simulink model "forwardsim6"  (R2019b)
settings: Solver=FixedStepAuto  StartTime=0.0  StopTime=21.75  FixedStep=1e-2  RelTol=1e-3
undefined symbols (not defined in the file or in its folder): auxdata, DiscIntNeverNeededParam, Earth, forwardsim, struct2bus, WGS84
libraries: aerolibasang x3, aerolibconvert2 x2, sharedutil x2, aerolib6dof2 x1, aerolibatmos2 x1, aerolibgravity2 x1
settings Model: Creator=kieran  LastModifiedBy=kieran

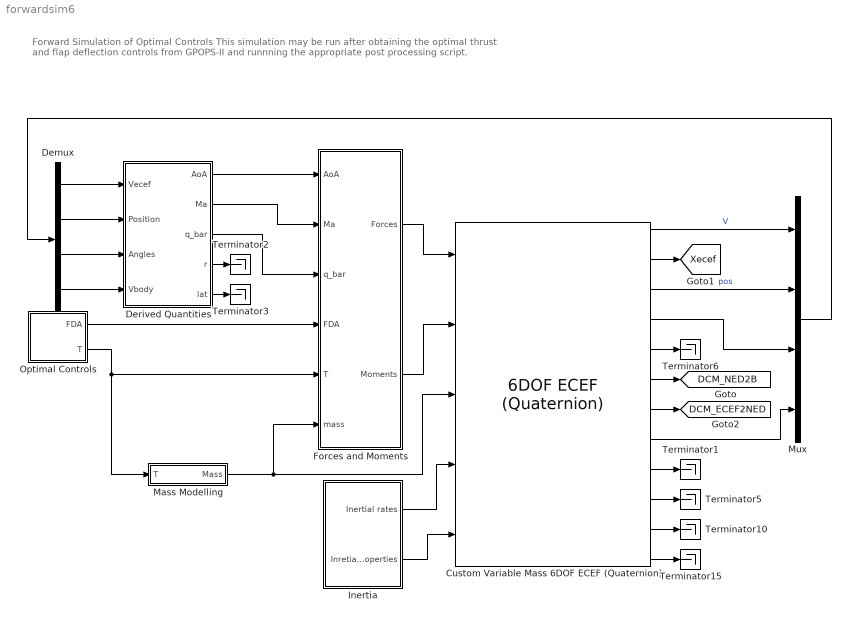
== system forwardsim6 ==
  note: Forward Simulation of Optimal Controls
      | This simulation may be run after obtaining the optimal thrust and flap deflection controls from GPOPS-II and runnning the appropriate post processing script.
  Custom Variable Mass 6DOF ECEF (Quaternion) : aerolib6dof2/6DOF ECEF (Quaternion)  units=Metric (MKS)  mtype=Custom Variable  xg_0=forwardsim.pos0  Vm_0=forwardsim.vel0  eul_0=forwardsim.EO0  pm_0=forwardsim.rot0  mass_0=mass  mass_e=0.5  mass_f=2.0  inertia=inertia  inertia_e=eye(3)  inertia_f=2*eye(3)  vre_flag=off  abi_flag=off  ptype=Earth (WGS84)  R=6378137  F=1/298.257223563  w_E=7292115e-11  angle_in=Internal  LG0=0  quat_statename=''  pm_statename=''  Vm_statename=''  posECEF_statename=''  posECI_statename=''  LG_statename=''  mass_statename=''
      settings: SourceProductName=Aerospace Blockset  SourceProductBaseCode=AE
  Demux : Demux
  Derived Quantities : Subsystem
  Forces and Moments : Subsystem
  Inertia : Subsystem
  Mass Modelling : Subsystem
  Mux : Mux
  Optimal Controls : Subsystem
  Terminator{1..3,5..6,10,15} (7 alike) : Terminator
  tag scope: DCM_ECEF2NED=global, DCM_NED2B=global, Xecef=global
  wires:
  Optimal Controls/2(T) -> Mass Modelling/1(T), Forces and Moments/5(T)
  Mux/1 -> Demux/1
  Inertia/2(Inretial Properties) -> Custom Variable Mass 6DOF ECEF (Quaternion)/5
  Inertia/1(Inertial rates) -> Custom Variable Mass 6DOF ECEF (Quaternion)/4
  Optimal Controls/1(FDA) -> Forces and Moments/4(FDA)
  Mass Modelling/1(Mass) -> Forces and Moments/6(mass), Custom Variable Mass 6DOF ECEF (Quaternion)/3
  Forces and Moments/2(Moments) -> Custom Variable Mass 6DOF ECEF (Quaternion)/2
  Forces and Moments/1(Forces) -> Custom Variable Mass 6DOF ECEF (Quaternion)/1
  Custom Variable Mass 6DOF ECEF (Quaternion)/7 -> [DCM_ECEF2NED]
  Custom Variable Mass 6DOF ECEF (Quaternion)/6 -> [DCM_NED2B]
  Custom Variable Mass 6DOF ECEF (Quaternion)/9 -> Terminator1/1
  Custom Variable Mass 6DOF ECEF (Quaternion)/10 -> Terminator5/1
  Custom Variable Mass 6DOF ECEF (Quaternion)/5 -> Terminator6/1
  Custom Variable Mass 6DOF ECEF (Quaternion)/11 -> Terminator10/1
  Custom Variable Mass 6DOF ECEF (Quaternion)/12 -> Terminator15/1
  Custom Variable Mass 6DOF ECEF (Quaternion)/3 -> Mux/2  "pos"
  Custom Variable Mass 6DOF ECEF (Quaternion)/1 -> Mux/1  "V"
  Custom Variable Mass 6DOF ECEF (Quaternion)/8 -> Mux/4
  Custom Variable Mass 6DOF ECEF (Quaternion)/4 -> Mux/3
  Demux/1 -> Derived Quantities/1(Vecef)
  Demux/2 -> Derived Quantities/2(Position)
  Demux/3 -> Derived Quantities/3(Angles)
  Demux/4 -> Derived Quantities/4(Vbody)
  Derived Quantities/1(AoA) -> Forces and Moments/1(AoA)
  Derived Quantities/2(Ma) -> Forces and Moments/2(Ma)
  Derived Quantities/3(q_bar) -> Forces and Moments/3(q_bar)
  Custom Variable Mass 6DOF ECEF (Quaternion)/2 -> [Xecef]
  Derived Quantities/5(lat) -> Terminator3/1
  Derived Quantities/4(r) -> Terminator2/1

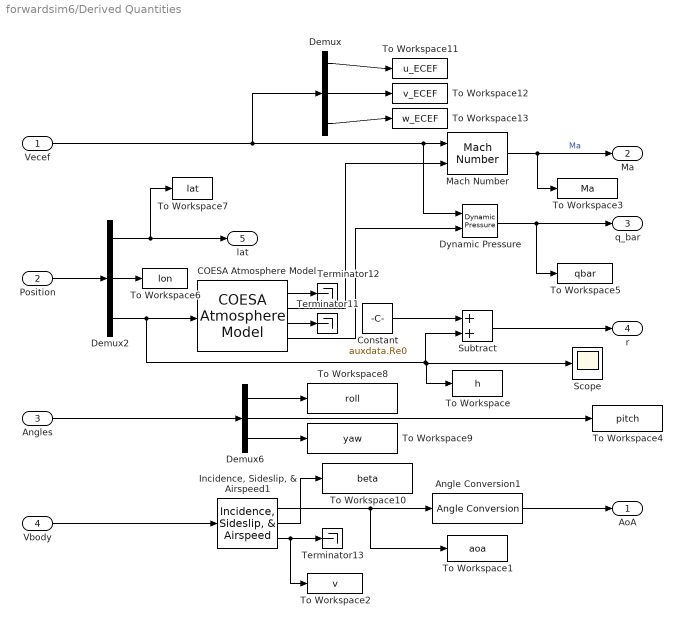
== system forwardsim6/Derived Quantities ==
  Vecef : Inport
  Position : Inport  Port=2
  Angles : Inport  Port=3
  Vbody : Inport  Port=4
  Angle Conversion1 : aerolibconvert2/Angle Conversion  IU=rad  OU=deg
  COESA Atmosphere Model : aerolibatmos2/COESA Atmosphere Model  units=Metric (MKS)  spec=1976 COESA-extended U.S. Standard Atmosphere  model=Profile  profile_var=High temperature  profile_percent=1%  profile_alt=5 km (16404 ft)  envelope_var=High temperature  envelope_percent=1%  action=Warning
  Constant : Constant  Value=auxdata.Re0
  Demux : Demux  Outputs=3
  Demux2 : Demux  Outputs=3
  Demux6 : Demux  Outputs=3
  Dynamic Pressure : aerolibasang/Dynamic Pressure
  "Incidence, Sideslip, & Airspeed1" : aerolibasang/Incidence, Sideslip, & Airspeed
      settings: SourceProductName=Aerospace Blockset
  Mach Number : aerolibasang/Mach Number
      settings: SourceProductName=Aerospace Blockset  SourceProductBaseCode=AE
  Scope : Scope
  Subtract : Sum
  Terminator11 : Terminator
  Terminator12 : Terminator
  Terminator13 : Terminator
  To Workspace : ToWorkspace  VariableName=h  SaveFormat=Timeseries  SampleTime=-1
  To Workspace1 : ToWorkspace  VariableName=aoa  SaveFormat=Timeseries  SampleTime=-1
  To Workspace10 : ToWorkspace  VariableName=beta  SaveFormat=Timeseries  SampleTime=-1
  To Workspace11 : ToWorkspace  VariableName=u_ECEF  SaveFormat=Timeseries  SampleTime=-1
  To Workspace12 : ToWorkspace  VariableName=v_ECEF  SaveFormat=Timeseries  SampleTime=-1
  To Workspace13 : ToWorkspace  VariableName=w_ECEF  SaveFormat=Timeseries  SampleTime=-1
  To Workspace2 : ToWorkspace  VariableName=v  SaveFormat=Timeseries  SampleTime=-1
  To Workspace3 : ToWorkspace  VariableName=Ma  SaveFormat=Timeseries  SampleTime=-1
  To Workspace4 : ToWorkspace  VariableName=pitch  SaveFormat=Timeseries  SampleTime=-1
  To Workspace5 : ToWorkspace  VariableName=qbar  SaveFormat=Timeseries  SampleTime=-1
  To Workspace6 : ToWorkspace  VariableName=lon  SaveFormat=Timeseries  SampleTime=-1
  To Workspace7 : ToWorkspace  VariableName=lat  SaveFormat=Timeseries  SampleTime=-1
  To Workspace8 : ToWorkspace  VariableName=roll  SaveFormat=Timeseries  SampleTime=-1
  To Workspace9 : ToWorkspace  VariableName=yaw  SaveFormat=Timeseries  SampleTime=-1
  AoA : Outport
  Ma : Outport  Port=2
  q_bar : Outport  Port=3
  r : Outport  Port=4
  lat : Outport  Port=5
  wires:
  Demux2/2 -> To Workspace6/1
  COESA Atmosphere Model/3 -> Terminator11/1
  Vecef/1 -> Demux/1, Dynamic Pressure/1, Mach Number/1
  "Incidence, Sideslip, & Airspeed1"/2 -> To Workspace10/1
  COESA Atmosphere Model/1 -> Terminator12/1
  Demux2/3 -> To Workspace/1, Scope/1, Subtract/2, COESA Atmosphere Model/1
  Demux2/1 -> To Workspace7/1, lat/1
  COESA Atmosphere Model/2 -> Mach Number/2
  Demux6/3 -> To Workspace9/1
  Angles/1 -> Demux6/1
  Subtract/1 -> r/1
  COESA Atmosphere Model/4 -> Dynamic Pressure/2
  "Incidence, Sideslip, & Airspeed1"/3 -> Terminator13/1, To Workspace2/1
  "Incidence, Sideslip, & Airspeed1"/1 -> To Workspace1/1, Angle Conversion1/1
  Vbody/1 -> "Incidence, Sideslip, & Airspeed1"/1
  Demux6/1 -> To Workspace8/1
  Position/1 -> Demux2/1
  Angle Conversion1/1 -> AoA/1
  Mach Number/1 -> To Workspace3/1, Ma/1  "Ma"
  Dynamic Pressure/1 -> To Workspace5/1, q_bar/1
  Demux6/2 -> To Workspace4/1
  Constant/1 -> Subtract/1
  Demux/1 -> To Workspace11/1
  Demux/3 -> To Workspace13/1
  Demux/2 -> To Workspace12/1

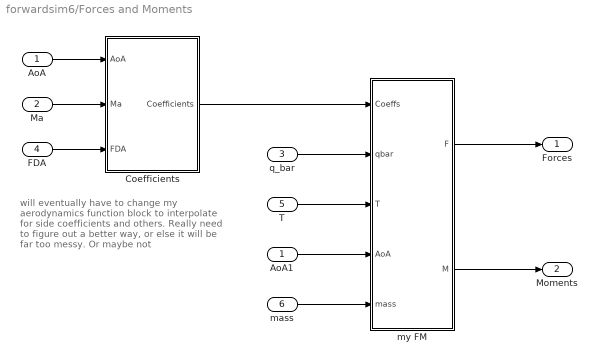
== system forwardsim6/Forces and Moments ==
  note: will eventually have to change my aerodynamics function block to interpolate for side coefficients and others. Really need to figure out a better way, or else it will be far too messy.
      |
      | Or maybe not
  AoA : Inport
  Ma : Inport  Port=2
  q_bar : Inport  Port=3
  FDA : Inport  Port=4
  T : Inport  Port=5
  mass : Inport  Port=6
  AoA1 : InportShadow
  Coefficients : Subsystem
  my FM : Subsystem
  Forces : Outport
  Moments : Outport  Port=2
  wires:
  Ma/1 -> Coefficients/2(Ma)
  FDA/1 -> Coefficients/3(FDA)
  Coefficients/1(Coefficients) -> my FM/1(Coeffs)
  q_bar/1 -> my FM/2(qbar)
  T/1 -> my FM/3(T)
  AoA/1 -> Coefficients/1(AoA)
  my FM/1(F) -> Forces/1
  AoA1/1 -> my FM/4(AoA)
  mass/1 -> my FM/5(mass)
  my FM/2(M) -> Moments/1

== system forwardsim6/Inertia ==
  Constant : Constant  Value=auxdata.MOI
  Constant3 : Constant  Commented=on  Value=auxdata.Iyy
  Inertia : Subsystem  Commented=on
  Inertial Rates : Subsystem
  Inertial rates : Outport
  Inretial Properties : Outport  Port=2
  wires:
  Constant3/1 -> Inertia/1(In1)
  Inertial Rates/1(Out1) -> Inertial rates/1
  Constant/1 -> Inretial Properties/1

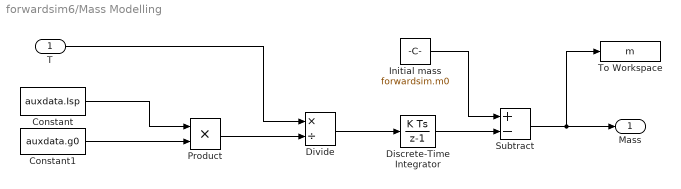
== system forwardsim6/Mass Modelling ==
  T : Inport
  Constant : Constant  Value=auxdata.Isp
  Constant1 : Constant  Value=auxdata.g0
  Discrete-Time Integrator : DiscreteIntegrator  SampleTime=-1  ICPrevOutput=DiscIntNeverNeededParam  ICPrevScaledInput=DiscIntNeverNeededParam
  Divide : Product  Inputs=*/
  Initial mass : Constant  Value=forwardsim.m0
  Product : Product
  Subtract : Sum  Inputs=+-
  To Workspace : ToWorkspace  VariableName=m  SaveFormat=Timeseries  SampleTime=-1
  Mass : Outport
  wires:
  Constant1/1 -> Product/2
  Divide/1 -> Discrete-Time Integrator/1
  Product/1 -> Divide/2
  Constant/1 -> Product/1
  Subtract/1 -> To Workspace/1, Mass/1
  Discrete-Time Integrator/1 -> Subtract/2
  Initial mass/1 -> Subtract/1
  T/1 -> Divide/1

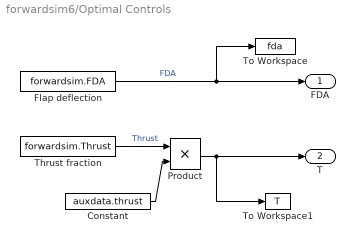
== system forwardsim6/Optimal Controls ==
  Constant : Constant  Value=auxdata.thrust
  Flap deflection : FromWorkspace  VariableName=forwardsim.FDA  SampleTime=0
  Product : Product
  Thrust fraction : FromWorkspace  VariableName=forwardsim.Thrust  SampleTime=0
  To Workspace : ToWorkspace  VariableName=fda  SaveFormat=Timeseries  SampleTime=-1
  To Workspace1 : ToWorkspace  VariableName=T  SaveFormat=Timeseries  SampleTime=-1
  FDA : Outport
  T : Outport  Port=2
  wires:
  Flap deflection/1 -> To Workspace/1, FDA/1  "FDA"
  Constant/1 -> Product/2
  Product/1 -> T/1, To Workspace1/1
  Thrust fraction/1 -> Product/1  "Thrust"

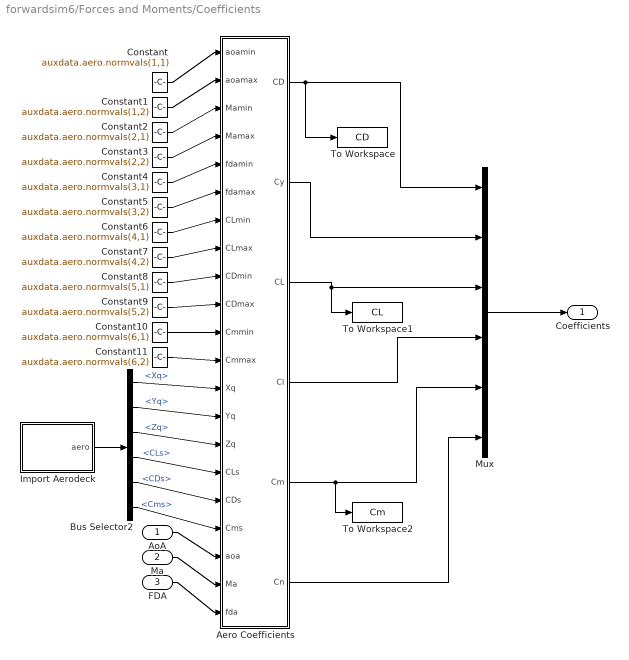
== system forwardsim6/Forces and Moments/Coefficients ==
  AoA : Inport
  Ma : Inport  Port=2
  FDA : Inport  Port=3
  Aero Coefficients : MATLAB Function  TreatAsAtomicUnit=on
  Bus Selector2 : BusSelector  OutputSignals=Xq,Yq,Zq,CLs,CDs,Cms
  Constant : Constant  Value=auxdata.aero.normvals(1,1)
  Constant1 : Constant  Value=auxdata.aero.normvals(1,2)
  Constant10 : Constant  Value=auxdata.aero.normvals(6,1)
  Constant11 : Constant  Value=auxdata.aero.normvals(6,2)
  Constant2 : Constant  Value=auxdata.aero.normvals(2,1)
  Constant3 : Constant  Value=auxdata.aero.normvals(2,2)
  Constant4 : Constant  Value=auxdata.aero.normvals(3,1)
  Constant5 : Constant  Value=auxdata.aero.normvals(3,2)
  Constant6 : Constant  Value=auxdata.aero.normvals(4,1)
  Constant7 : Constant  Value=auxdata.aero.normvals(4,2)
  Constant8 : Constant  Value=auxdata.aero.normvals(5,1)
  Constant9 : Constant  Value=auxdata.aero.normvals(5,2)
  Import Aerodeck : MATLAB Function  InitFcn=struct2bus(auxdata.aero,'aerodeck')  TreatAsAtomicUnit=on
  Mux : Mux  Inputs=6
  To Workspace : ToWorkspace  VariableName=CD  SaveFormat=Timeseries  SampleTime=-1
  To Workspace1 : ToWorkspace  VariableName=CL  SaveFormat=Timeseries  SampleTime=-1
  To Workspace2 : ToWorkspace  VariableName=Cm  SaveFormat=Timeseries  SampleTime=-1
  Coefficients : Outport
  wires:
  Bus Selector2/1 -> Aero Coefficients/13(Xq)  "<Xq>"
  Constant11/1 -> Aero Coefficients/12(Cmmax)
  Bus Selector2/3 -> Aero Coefficients/15(Zq)  "<Zq>"
  Aero Coefficients/5(Cm) -> Mux/5, To Workspace2/1
  Mux/1 -> Coefficients/1
  Aero Coefficients/2(Cy) -> Mux/2
  Constant3/1 -> Aero Coefficients/4(Mamax)
  Constant1/1 -> Aero Coefficients/2(aoamax)
  Constant5/1 -> Aero Coefficients/6(fdamax)
  Constant4/1 -> Aero Coefficients/5(fdamin)
  Constant8/1 -> Aero Coefficients/9(CDmin)
  AoA/1 -> Aero Coefficients/19(aoa)
  Constant7/1 -> Aero Coefficients/8(CLmax)
  FDA/1 -> Aero Coefficients/21(fda)
  Bus Selector2/5 -> Aero Coefficients/17(CDs)  "<CDs>"
  Aero Coefficients/3(CL) -> Mux/3, To Workspace1/1
  Constant2/1 -> Aero Coefficients/3(Mamin)
  Constant10/1 -> Aero Coefficients/11(Cmmin)
  Constant9/1 -> Aero Coefficients/10(CDmax)
  Aero Coefficients/1(CD) -> Mux/1, To Workspace/1
  Constant6/1 -> Aero Coefficients/7(CLmin)
  Import Aerodeck/1(aero) -> Bus Selector2/1
  Bus Selector2/6 -> Aero Coefficients/18(Cms)  "<Cms>"
  Ma/1 -> Aero Coefficients/20(Ma)
  Aero Coefficients/6(Cn) -> Mux/6
  Bus Selector2/4 -> Aero Coefficients/16(CLs)  "<CLs>"
  Constant/1 -> Aero Coefficients/1(aoamin)
  Bus Selector2/2 -> Aero Coefficients/14(Yq)  "<Yq>"
  Aero Coefficients/4(Cl) -> Mux/4

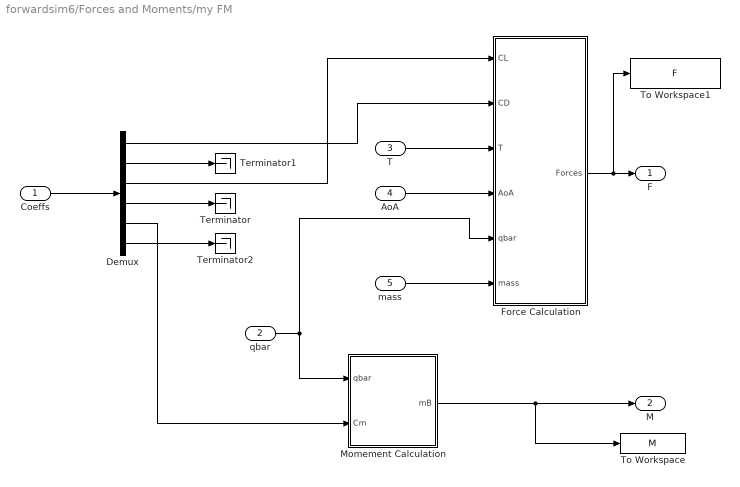
== system forwardsim6/Forces and Moments/my FM ==
  Coeffs : Inport
  qbar : Inport  Port=2
  T : Inport  Port=3
  AoA : Inport  Port=4
  mass : Inport  Port=5
  Demux : Demux  Outputs=6
  Force Calculation : Subsystem
  Momement Calculation : Subsystem
  Terminator : Terminator
  Terminator1 : Terminator
  Terminator2 : Terminator
  To Workspace : ToWorkspace  VariableName=M  SaveFormat=Timeseries  SampleTime=-1
  To Workspace1 : ToWorkspace  VariableName=F  SaveFormat=Timeseries  SampleTime=-1
  F : Outport
  M : Outport  Port=2
  wires:
  Coeffs/1 -> Demux/1
  Demux/5 -> Momement Calculation/2(Cm)
  Demux/4 -> Terminator/1
  Demux/2 -> Terminator1/1
  Demux/6 -> Terminator2/1
  qbar/1 -> Force Calculation/5(qbar), Momement Calculation/1(qbar)
  T/1 -> Force Calculation/3(T)
  AoA/1 -> Force Calculation/4(AoA)
  Force Calculation/1(Forces) -> To Workspace1/1, F/1
  Momement Calculation/1(mB) -> To Workspace/1, M/1
  Demux/1 -> Force Calculation/2(CD)
  Demux/3 -> Force Calculation/1(CL)
  mass/1 -> Force Calculation/6(mass)

== system forwardsim6/Inertia/Inertia ==
  In1 : Inport
  Constant : Constant  Value=0
  Constant1 : Constant  Value=0
  Create 3x3 Matrix : sharedutil/Create 3x3 Matrix  aMode=aMode
  Out1 : Outport
  wires:
  Create 3x3 Matrix/1 -> Out1/1
  Constant/1 -> Create 3x3 Matrix/2, Create 3x3 Matrix/3, Create 3x3 Matrix/4
  Constant1/1 -> Create 3x3 Matrix/8, Create 3x3 Matrix/6, Create 3x3 Matrix/7
  In1/1 -> Create 3x3 Matrix/1, Create 3x3 Matrix/9, Create 3x3 Matrix/5

== system forwardsim6/Inertia/Inertial Rates ==
  Constant1 : Constant  Value=0
  Create 3x3 Matrix : sharedutil/Create 3x3 Matrix  aMode=aMode
  Out1 : Outport
  wires:
  Create 3x3 Matrix/1 -> Out1/1
  Constant1/1 -> Create 3x3 Matrix/1, Create 3x3 Matrix/2, Create 3x3 Matrix/3, Create 3x3 Matrix/4, Create 3x3 Matrix/9, Create 3x3 Matrix/8, Create 3x3 Matrix/7, Create 3x3 Matrix/6, Create 3x3 Matrix/5

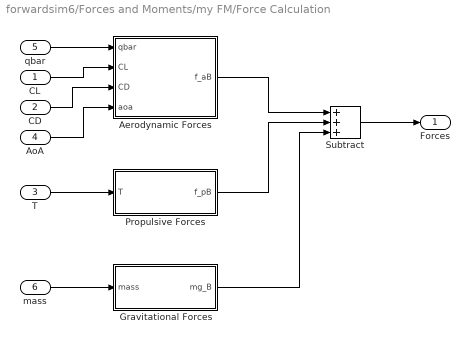
== system forwardsim6/Forces and Moments/my FM/Force Calculation ==
  CL : Inport
  CD : Inport  Port=2
  T : Inport  Port=3
  AoA : Inport  Port=4
  qbar : Inport  Port=5
  mass : Inport  Port=6
  Aerodynamic Forces : Subsystem
  Gravitational Forces : Subsystem
  Propulsive Forces : Subsystem
  Subtract : Sum  Inputs=+++
  Forces : Outport
  wires:
  AoA/1 -> Aerodynamic Forces/4(aoa)
  Aerodynamic Forces/1(f_aB) -> Subtract/1
  Propulsive Forces/1(f_pB) -> Subtract/2
  qbar/1 -> Aerodynamic Forces/1(qbar)
  CL/1 -> Aerodynamic Forces/2(CL)
  CD/1 -> Aerodynamic Forces/3(CD)
  T/1 -> Propulsive Forces/1(T)
  mass/1 -> Gravitational Forces/1(mass)
  Subtract/1 -> Forces/1
  Gravitational Forces/1(mg_B) -> Subtract/3

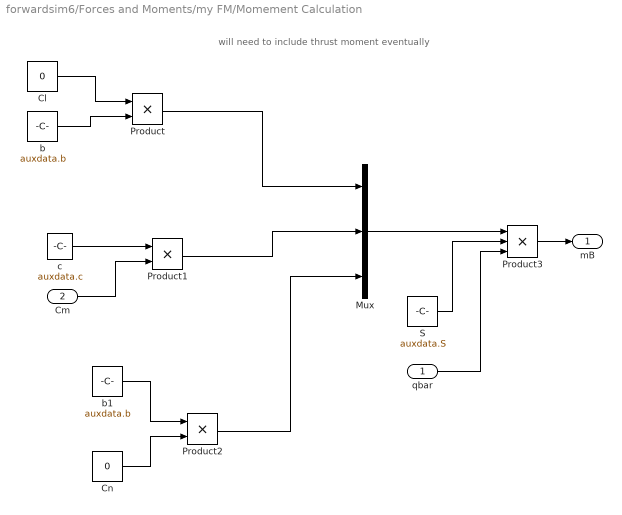
== system forwardsim6/Forces and Moments/my FM/Momement Calculation ==
  note: will need to include thrust moment eventually
  qbar : Inport
  Cm : Inport  Port=2
  Cl : Constant  Value=0
  Cn : Constant  Value=0
  Mux : Mux  Inputs=3
  Product : Product
  Product1 : Product
  Product2 : Product
  Product3 : Product  Inputs=3
  S : Constant  Value=auxdata.S
  b : Constant  Value=auxdata.b
  b1 : Constant  Value=auxdata.b
  c : Constant  Value=auxdata.c
  mB : Outport
  wires:
  Cn/1 -> Product2/2
  b1/1 -> Product2/1
  Cl/1 -> Product/1
  b/1 -> Product/2
  c/1 -> Product1/1
  Cm/1 -> Product1/2
  Product1/1 -> Mux/2
  Product/1 -> Mux/1
  Product2/1 -> Mux/3
  Mux/1 -> Product3/1
  Product3/1 -> mB/1
  S/1 -> Product3/2
  qbar/1 -> Product3/3

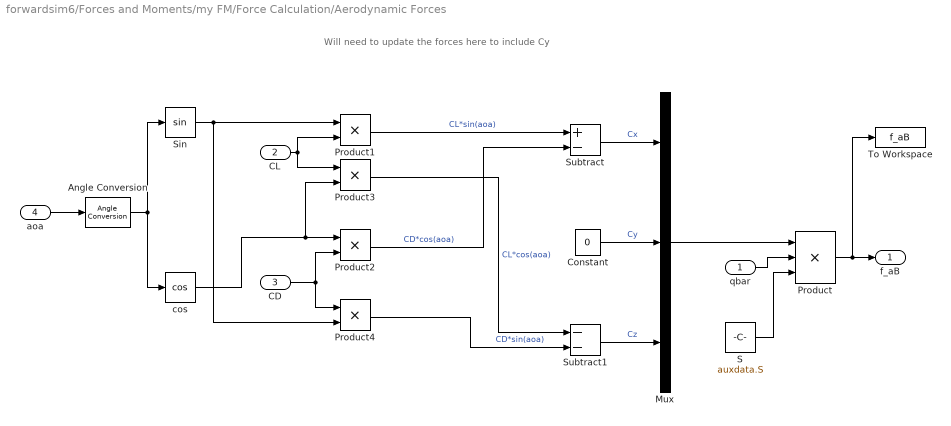
== system forwardsim6/Forces and Moments/my FM/Force Calculation/Aerodynamic Forces ==
  note: Will need to update the forces here to include Cy
  qbar : Inport
  CL : Inport  Port=2
  CD : Inport  Port=3
  aoa : Inport  Port=4
  Angle Conversion : aerolibconvert2/Angle Conversion  IU=deg  OU=rad
  Constant : Constant  Value=0
  Mux : Mux  Inputs=3
  Product : Product  Inputs=3
  Product{1..4} (4 alike) : Product
  S : Constant  Value=auxdata.S
  Sin : Trigonometry
  Subtract : Sum  Inputs=+-
  Subtract1 : Sum  Inputs=--
  To Workspace : ToWorkspace  VariableName=f_aB  SaveFormat=Timeseries  SampleTime=-1
  cos : Trigonometry  Operator=cos
  f_aB : Outport
  wires:
  Product/1 -> To Workspace/1, f_aB/1
  Mux/1 -> Product/1
  qbar/1 -> Product/2
  S/1 -> Product/3
  CL/1 -> Product3/1, Product1/2
  Sin/1 -> Product4/2, Product1/1
  CD/1 -> Product2/2, Product4/1
  cos/1 -> Product2/1, Product3/2
  Product4/1 -> Subtract1/2  "CD*sin(aoa)"
  Product2/1 -> Subtract/2  "CD*cos(aoa)"
  Product3/1 -> Subtract1/1  "CL*cos(aoa)"
  Product1/1 -> Subtract/1  "CL*sin(aoa)"
  Subtract1/1 -> Mux/3  "Cz"
  Subtract/1 -> Mux/1  "Cx"
  Constant/1 -> Mux/2  "Cy"
  aoa/1 -> Angle Conversion/1
  Angle Conversion/1 -> cos/1, Sin/1

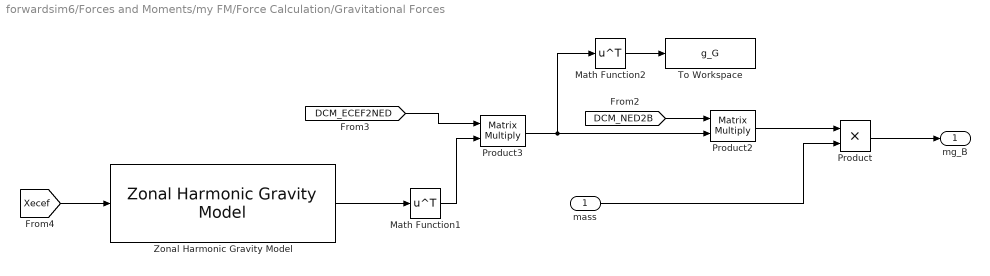
== system forwardsim6/Forces and Moments/my FM/Force Calculation/Gravitational Forces ==
  mass : Inport
  Math Function1 : Math  Operator=transpose  SignedPower=off  SaturateOnIntegerOverflow=on
  Math Function2 : Math  Operator=transpose  SignedPower=off  SaturateOnIntegerOverflow=on
  Product : Product
  Product2 : Product  Multiplication=Matrix(*)
  Product3 : Product  Multiplication=Matrix(*)
  To Workspace : ToWorkspace  VariableName=g_G  SaveFormat=Timeseries  SampleTime=-1
  Zonal Harmonic Gravity Model : aerolibgravity2/Zonal Harmonic Gravity Model  units=Metric (MKS)  degree=4  action=Warning  ptype=Earth  R=6378136.3  GM=398600441500000  jvalue=[1.0826269e-03 -2.5323000e-06 -1.6204000e-06]
      settings: SourceProductName=Aerospace Blockset  SourceProductBaseCode=AE
  mg_B : Outport
  wires:
  mass/1 -> Product/2
  [DCM_NED2B] -> Product2/1
  Product/1 -> mg_B/1
  [DCM_ECEF2NED] -> Product3/1
  Zonal Harmonic Gravity Model/1 -> Math Function1/1
  Math Function1/1 -> Product3/2
  [Xecef] -> Zonal Harmonic Gravity Model/1
  Product3/1 -> Math Function2/1, Product2/2
  Math Function2/1 -> To Workspace/1
  Product2/1 -> Product/1

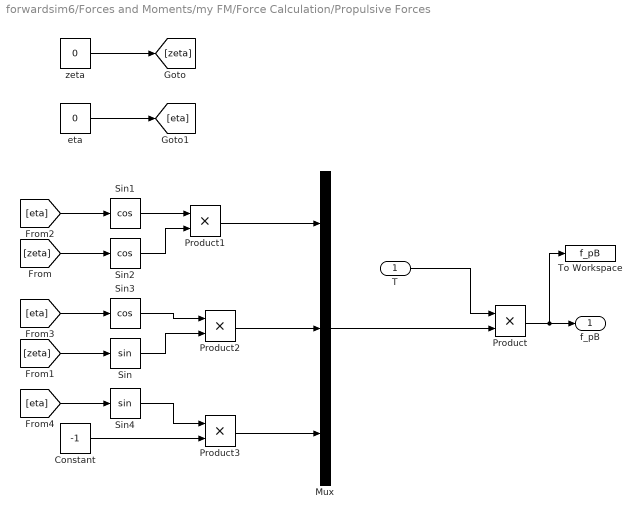
== system forwardsim6/Forces and Moments/my FM/Force Calculation/Propulsive Forces ==
  T : Inport
  Constant : Constant  Value=-1
  Mux : Mux  Inputs=3
  Product{,1..3} (4 alike) : Product
  Sin : Trigonometry
  Sin1 : Trigonometry  Operator=cos
  Sin2 : Trigonometry  Operator=cos
  Sin3 : Trigonometry  Operator=cos
  Sin4 : Trigonometry
  To Workspace : ToWorkspace  VariableName=f_pB  SaveFormat=Timeseries  SampleTime=-1
  eta : Constant  Value=0
  zeta : Constant  Value=0
  f_pB : Outport
  wires:
  T/1 -> Product/1
  Mux/1 -> Product/2
  zeta/1 -> [zeta]
  eta/1 -> [eta]
  Sin1/1 -> Product1/1
  Sin2/1 -> Product1/2
  Product1/1 -> Mux/1
  [eta] -> Sin3/1
  [zeta] -> Sin/1
  Sin3/1 -> Product2/1
  Sin/1 -> Product2/2
  Product2/1 -> Mux/2
  [eta] -> Sin4/1
  Product3/1 -> Mux/3
  Sin4/1 -> Product3/1
  Constant/1 -> Product3/2
  [zeta] -> Sin2/1
  [eta] -> Sin1/1
  Product/1 -> To Workspace/1, f_pB/1

== matlab function forwardsim6/Forces and Moments/Coefficients/Aero Coefficients ==
  data: aoamin input; aoamax input; Mamin input; Mamax input; fdamin input; fdamax input; CLmin input; CLmax input; CDmin input; CDmax input; Cmmin input; Cmmax input; CD output; Cy output; Xq input; Yq input; Zq input; CLs input; CDs input; Cms input; CL output; Cl output; aoa input; Ma input; fda input; Cm output; Cn output
function [CD,Cy,CL,Cl,Cm,Cn] = GetAero(aoamin,aoamax,Mamin,Mamax,...
    fdamin,fdamax,CLmin,CLmax,CDmin,CDmax,Cmmin,Cmmax,...
    Xq,Yq,Zq,CLs,CDs,Cms,aoa,Ma,fda)

Cy  = 0;
Cl  = 0;
Cn  = 0;

% normalise inputs
aoa = (aoa-aoamin)./(aoamax-aoamin);
Ma  = (Ma -Mamin)./(Mamax-Mamin);
fda = (fda-fdamin)./(fdamax-fdamin);

CL  = interp3(Xq,Yq,Zq,CLs,aoa,Ma,fda,'spline');
CD  = interp3(Xq,Yq,Zq,CDs,aoa,Ma,fda,'spline');
Cm  = interp3(Xq,Yq,Zq,Cms,aoa,Ma,fda,'spline');

% De-normalise coefficients
CL  = CL.*(CLmax-CLmin) + CLmin;
CD  = CD.*(CDmax-CDmin) + CDmin;
Cm  = Cm.*(Cmmax-Cmmin) + Cmmin;

end

== matlab function forwardsim6/Forces and Moments/Coefficients/Import Aerodeck ==
  data: aero output Bus: aerodeck
function aero = fcn

eml.extrinsic('evalin');

aero = evalin('base', 'auxdata.aero');
